simulink model "ACDCMG_sim8"  (R2022a)
settings: Solver=FixedStepAuto  StartTime=0.0  StopTime=0.5  FixedStep=Ts  MaxStep=1e-2  RelTol=1e-3
InitFcn:
  | Set_parameters_R2018
values from neighbouring files (symbols this model uses):
  D_invs = 0.05    [Set_parameters_R2018.m]
  dis11 = 3    [Set_parameters_R2018.m]
  dis12 = 3    [Set_parameters_R2018.m]
  dis2 = 0.2    [Set_parameters_R2018.m]
  dis3 = 0.15    [Set_parameters_R2018.m]
  dis4 = 0.2    [Set_parameters_R2018.m]
  dis5 = 0.25    [Set_parameters_R2018.m]
  dis6 = 0.1    [Set_parameters_R2018.m]
  Fnom = 60    [Set_parameters_R2018.m]
  H_invs = 6    [Set_parameters_R2018.m]
  max_min = 1    [Set_parameters_R2018.m]
  P_Load_3 = S_Load_3* PF_Load_3    (= 7650)    [Set_parameters_R2018.m]
  P_nom_inv = 3e3    (= 3000)    [Set_parameters_R2018.m]
  Pnom_T1 = 1.5e6    (= 1500000)    [Set_parameters_R2018.m]
  Pnom_T2 = 1.5e6    (= 1500000)    [Set_parameters_R2018.m]
  Pnom_T3 = 4e6    (= 4000000)    [Set_parameters_R2018.m]
  Ql_Load_3 = S_Load_3 * sin(acos(PF_Load_3))    [Set_parameters_R2018.m]
  R_Load_9 = (Vnom_prim * 1.35)^2 / P_Load_9    (= 1084.6153125)    [Set_parameters_R2018.m]
  R_Load_DC = Vnom_DC^2/ P_Load_DC    (= 45)    [Set_parameters_R2018.m]
  Rl = 0.17    [Set_parameters_R2018.m]
  Rls = 0.013    [Set_parameters_R2018.m]
  Ts = Ts_Power    (= 6.94444444444e-06)    [Set_parameters_R2018.m]
  Ts_Control = 6*Ts_Power    (= 4.16666666667e-05)    [Set_parameters_R2018.m]
  Ts_Inv = 0.07    [Set_parameters_R2018.m]
  Ts_Power = 1/(24*Fnom)/100    (= 6.94444444444e-06)    [Set_parameters_R2018.m]
  Ts_PV = 0.05    [Set_parameters_R2018.m]
  V1_LL_T3 = 69e3    (= 69000)    [Set_parameters_R2018.m]
  Vmin_mppt = 100    [Set_parameters_R2018.m]
  Vnom_DC = 300    [Set_parameters_R2018.m]
  Vnom_Diesel = 2.4e3    (= 2400)    [Set_parameters_R2018.m]
  Vnom_prim = 13.8e3    (= 13800)    [Set_parameters_R2018.m]
  Vnom_sec = 220    [Set_parameters_R2018.m]
  Vnom_ter_AC_DC = 150    [Set_parameters_R2018.m]
  Xl = 0.3    [Set_parameters_R2018.m]
  Xls = 0.93e-3    (= 0.00093)    [Set_parameters_R2018.m]
undefined symbols (not defined in the file or in its folder): D1, dEgdT, Delta, DiscIntNeverNeededParam, EgRef, fn, gcbh, Ion, k1, Lithium, Rsh_array5pc, sps_rtmsupport, Tref_K, VnInv, VT_ref
libraries: spsCurrentMeasurementLib x40, spsRMSLib x29, spsSeriesRLCBranchLib x23, spsVoltageMeasurementLib x21, spsMeanLib x14, spsThreePhaseVIMeasurementLib x14, powerlib_extras x13, spsThreePhaseSeriesRLCBranchLib x12, spsPower3phInstantaneousLib x10, spsBreakerLib x8, spsControlledVoltageSourceLib x8, spsPowerLib x8
(part 1 of 12)
settings Model: Creator=Leony  LastModifiedBy=dkh20
settings SolverCC: ZeroCrossAlgorithm=Adaptive  SolverResetMethod=Robust
settings DataIOCC: LimitDataPoints=on  SaveFormat=Array  ReturnWorkspaceOutputs=off
settings OptimizationCC: LifeSpan=inf
settings DebuggingCC: AlgebraicLoopMsg=none  UnderspecifiedInitializationDetection=Classic  MergeDetectMultiDrivingBlocksExec=none  IgnoredZcDiagnostic=none  SolverPrmCheckMsg=warning  UnconnectedInputMsg=warning  UnconnectedOutputMsg=warning  UnconnectedLineMsg=warning  AllowSymbolicDim=off  SFUnexpectedBacktrackingDiag=warning  SFNoUnconditionalDefaultTransitionDiag=warning  SFExecutionAtInitializationDiag=none  SFMachineParentedDataDiag=warning  ArithmeticOperatorsInVariantConditions=warning
settings HardwareCC: ProdBitPerPointer=32  ProdBitPerSizeT=32  ProdBitPerPtrDiffT=32  ProdLargestAtomicFloat=None  ProdIntDivRoundTo=Undefined  ProdEndianess=Unspecified  ProdWordSize=32  ProdHWDeviceType=32-bit Generic
settings ModelReferenceCC: PropagateSignalLabelsOutOfModel=off
settings SFSimCC: SimUseLocalCustomCode=off  CustomCodeUndefinedFunction=UseInterfaceOnly
settings RTWCC: RTWUseLocalCustomCode=off  DLArmComputeVersion=19.05
settings CodeAppCC: StateflowObjectComments=on
settings GRTTargetCC: TargetLangStandard=C89/C90 (ANSI)
settings ConfigComp: CovMetricSettings=dw  CovSaveCumulativeToWorkspaceVar=on  CovSaveSingleToWorkspaceVar=on  CovExternalEMLEnable=off
settings SimscapeCC: SimscapeNormalizeSystem=off

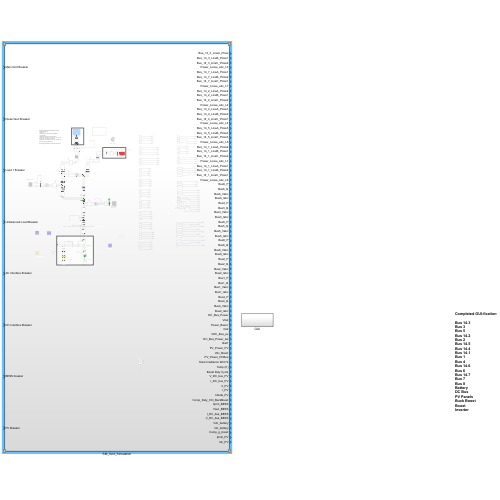
[thumbnail: Simulink's stored preview of the top-level diagram]
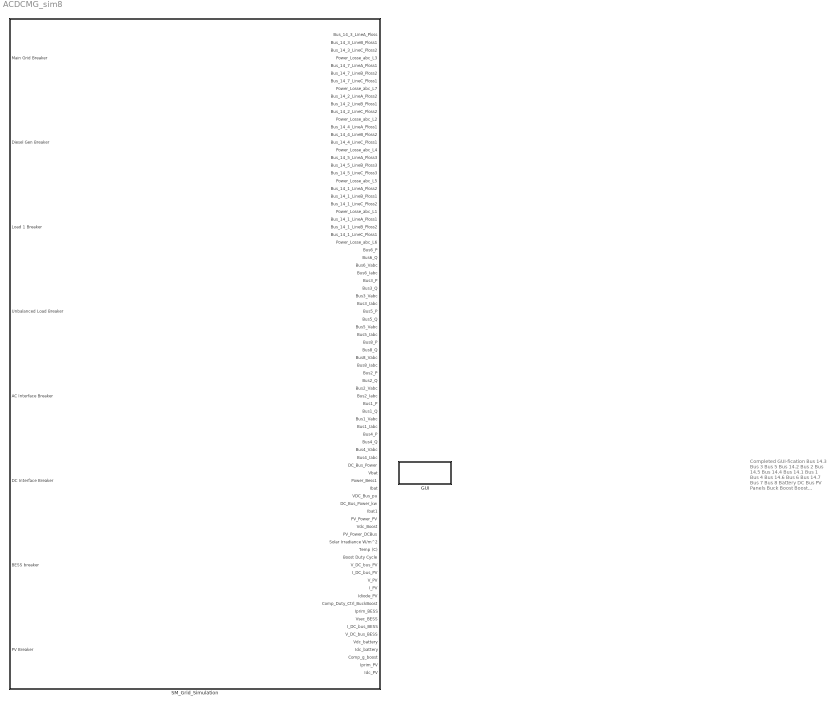
== system ACDCMG_sim8 ==
  note: Completed GUI-fication
      |
      | Bus 14.3
      | Bus 3
      | Bus 5
      | Bus 14.2
      | Bus 2
      | Bus 14.5
      | Bus 14.4
      | Bus 14.1
      | Bus 1
      | Bus 4
      | Bus 14.6
      | Bus 6
      | Bus 14.7
      | Bus 7
      | Bus 8
      | Battery
      | DC Bus
      | PV Panels
      | Buck Boost
      | Boost
      | Inverter
  GUI : Subsystem
  SM_Grid_Simulation : Subsystem

== system ACDCMG_sim8/GUI ==

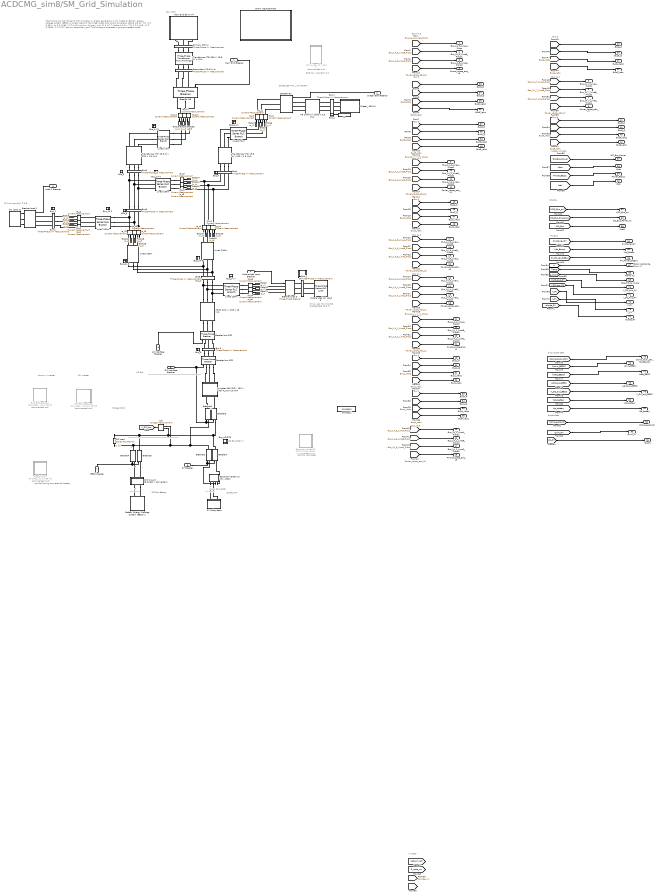
== system ACDCMG_sim8/SM_Grid_Simulation ==
  note: 9 kVA; cos (phi) = 0.85
      | Unbalanced 12.6 %
  note: +
  note: +
  note: Main Grid
  note: ---------------------------------------------------------------------------
  note: 2 kW
  note: +
  note: ---------------
  note: VF inverter
  note: DC Bus 300V V
  note: Microgrid DC
  note: Diesel_50 MVA _ Sim BusPV
  note: dump converter
  note: --------------------------------------------------------------------------------
  note: dummy converter
  note: dummy inverter
  note: ---------------
  note: -
  note: 12 kVA; cos (phi) = 0.6
  note: -
  note: DC Bus PV
  note: -
  note: DC Bus Battery
  note: The Hybrid AC /DC Microgrid (MG) includes:
      | 1- Diesel generators
      | 2- PV model
      | 3- Battery energy storage system (BESS)
      | 4- Linear loads
      | 5- Nonlinear loads such as arc furnace
      | 6- Cable 1/0 Cu, TW. R = 0.394 / XL = 0.1168 / Z = 0.411 per km. (Primary grid 13.8 kV)
      | 7- Cable 4/0 Cu , TW R = 0.198 / Xl = 0.1089 / Z = 0.227 per km (secondary grid)
      |
      | The microgrid operates in grid-connected mode.
  note: grid-following converter for battery
  note: +
  note: 320 kVA ; cos (phi) = 1
  note: AC Bus
  note: +
  note: -
  note: -
  note: inverter
  note: Bus 1
  note: Bus 14.4
  note: Bus 4
  note: Bus 5
  note: Bus 14.5
  note: Bus 14.6
  note: Bus 2
  note: Bus 3
  note: Bus 14.1
  note: Bus 14.2
  note: Bus 14.3
  note: Bus 8
  note: Bus 6
  note: DC_Bus
  note: PV_Bus
  note: buck boost data
  note: Bus 14.7
  note: battery_system
  note: boost data
  Main Grid Breaker : Inport
  Diesel Gen Breaker : Inport  Port=2
  Load 1 Breaker : Inport  Port=3
  Unbalanced Load Breaker : Inport  Port=4
  AC Interface Breaker : Inport  Port=5
  DC Interface Breaker : Inport  Port=6
  BESS breaker : Inport  Port=7
  PV Breaker : Inport  Port=8
    Ic_L{1,3..4,11} (4 alike) : spsCurrentMeasurementLib/Current Measurement  PhasorSimulation=off  OutputType=Complex  PSBequivalent=0
  AC  Load 11 : spsThreePhaseSeriesRLCLoadLib/Three-Phase Series RLC Load  LConnTagsString=A|B|C  Configuration=Y (grounded)  NominalVoltage=Vnom_sec  Vabc=[1e3 1e3 1e3]  Vabcp=[1e3 1e3 1e3]  NominalFrequency=Fnom  UnbalancedPower=off  ActivePower=P_Load_11  InductivePower=Ql_Load_11  CapacitivePower=0  Pabc=[10e3 9e3 11e3]  QLabc=[100 90 110]  QCabc=[100 90 110]  Pabcp=[10e3 9e3 11e3]  QLabcp=[100 90 110]  QCabcp=[100 90 110]  Measurements=None  LoadType=constant Z
  Battery Energy Storage System (BESS) 1 : Subsystem
      mask Display: image('Icons\Battery Energy Storage System (BESS).png');
  Boost -buck Bi-directional converter 1 : Subsystem
      mask Display: image(imread('Icons\DC_DC_Converter.jpg'));
  Boost -buck Bi-directional converter DC /CD 1 0.65 kW : Subsystem  Commented=on
      mask Display: image(imread('Icons\DC_DC_Converter.jpg'));
  "Boost converter 2 5 kHz - 300V " : Subsystem
      mask Display: image(imread('Icons\DC_DC_Converter.jpg'));
  "Boost converter DC /DC 2 5 kHz - 300V " : Subsystem  Commented=on
      mask Display: image(imread('Icons\DC_DC_Converter.jpg'));
  Breaker G1 : spsThreePhaseBreakerLib/Three-Phase Breaker  InitialState=closed  SwitchA=on  SwitchB=on  SwitchC=on  SwitchTimes="[4/60  10/60]"  External=on  BreakerResistance=0.001  SnubberResistance=1e6  SnubberCapacitance=inf  Measurements=None
  Breaker Load 1 : spsThreePhaseBreakerLib/Three-Phase Breaker  InitialState=closed  SwitchA=on  SwitchB=on  SwitchC=on  SwitchTimes="[4/60  10/60]"  External=on  BreakerResistance=0.001  SnubberResistance=1e6  SnubberCapacitance=inf  Measurements=None
  Breaker Load 3 : spsThreePhaseBreakerLib/Three-Phase Breaker  InitialState=closed  SwitchA=on  SwitchB=on  SwitchC=on  SwitchTimes="[4/60  10/60]"  External=on  BreakerResistance=0.001  SnubberResistance=1e6  SnubberCapacitance=inf  Measurements=None
  Breaker MG : spsThreePhaseBreakerLib/Three-Phase Breaker  InitialState=closed  SwitchA=on  SwitchB=on  SwitchC=on  SwitchTimes="[4/60  10/60]"  External=on  BreakerResistance=0.001  SnubberResistance=1e6  SnubberCapacitance=inf  Measurements=None
  Breaker bus DC1 : spsThreePhaseBreakerLib/Three-Phase Breaker  InitialState=closed  SwitchA=on  SwitchB=on  SwitchC=on  SwitchTimes="[4/60  10/60]"  External=on  BreakerResistance=0.001  SnubberResistance=1e6  SnubberCapacitance=inf  Measurements=None
  Breaker bus DC2 : spsThreePhaseBreakerLib/Three-Phase Breaker  InitialState=closed  SwitchA=on  SwitchB=on  SwitchC=on  SwitchTimes="[4/60  10/60]"  External=on  BreakerResistance=0.001  SnubberResistance=1e6  SnubberCapacitance=inf  Measurements=None
  Breaker{2..5} (4 alike) : spsBreakerLib/Breaker  InitialState=1  SwitchingTimes="[1/60  5/60]"  External=on  BreakerResistance=0.01  SnubberResistance=1e6  SnubberCapacitance=inf  Measurements=None  MoreParameters=on  NoBreakLoop=off
      settings: SourceProductBaseCode=PS
  Breaker6 : spsBreakerLib/Breaker  InitialState=0  SwitchingTimes="[1/60  5/60]"  External=on  BreakerResistance=0.01  SnubberResistance=1e6  SnubberCapacitance=inf  Measurements=None  MoreParameters=on  NoBreakLoop=off
      settings: SourceProductBaseCode=PS
  Breaker7 : spsBreakerLib/Breaker  InitialState=0  SwitchingTimes="[1/60  5/60]"  External=on  BreakerResistance=0.01  SnubberResistance=1e6  SnubberCapacitance=inf  Measurements=None  MoreParameters=on  NoBreakLoop=off
      settings: SourceProductBaseCode=PS
  Bus 1 : spsThreePhaseVIMeasurementLib/Three-Phase V-I Measurement  VoltageMeasurement=phase-to-phase  SetLabelV=on  LabelV=VabcLL_Bus_1  Vpu=off  VpuLL=off  CurrentMeasurement=yes  SetLabelI=on  LabelI=IabcLL_Bus_1  Ipu=off  Pbase=100e6  Vbase=25e3/sqrt(2)  OutputType=Complex  PhasorSimulation=off  PSBequivalent=0
  Bus 2 : spsThreePhaseVIMeasurementLib/Three-Phase V-I Measurement  VoltageMeasurement=phase-to-phase  SetLabelV=on  LabelV=VabcLL_Bus_2  Vpu=off  VpuLL=off  CurrentMeasurement=yes  SetLabelI=on  LabelI=IabcLL_Bus_2  Ipu=off  Pbase=100e6  Vbase=380/sqrt(2)  OutputType=Complex  PhasorSimulation=off  PSBequivalent=0
  Bus 7 : spsThreePhaseVIMeasurementLib/Three-Phase V-I Measurement  VoltageMeasurement=phase-to-phase  SetLabelV=on  LabelV=VabcLL_Bus_7  Vpu=off  VpuLL=off  CurrentMeasurement=yes  SetLabelI=on  LabelI=IabcLL_Bus_7  Ipu=off  Pbase=100e6  Vbase=380/sqrt(2)  OutputType=Complex  PhasorSimulation=off  PSBequivalent=0
  Bus 8 : spsThreePhaseVIMeasurementLib/Three-Phase V-I Measurement  VoltageMeasurement=phase-to-phase  SetLabelV=on  LabelV=VabcLL_Bus_8  Vpu=off  VpuLL=off  CurrentMeasurement=yes  SetLabelI=on  LabelI=IabcLL_Bus_8  Ipu=off  Pbase=100e6  Vbase=25e3  OutputType=Complex  PhasorSimulation=off  PSBequivalent=0
  Bus3 : spsThreePhaseVIMeasurementLib/Three-Phase V-I Measurement  VoltageMeasurement=phase-to-phase  SetLabelV=on  LabelV=VabcLL_Bus_3  Vpu=off  VpuLL=off  CurrentMeasurement=yes  SetLabelI=on  LabelI=IabcLL_Bus_3  Ipu=off  Pbase=100e6  Vbase=380/sqrt(2)  OutputType=Complex  PhasorSimulation=off  PSBequivalent=0
  Bus4 : spsThreePhaseVIMeasurementLib/Three-Phase V-I Measurement  VoltageMeasurement=phase-to-phase  SetLabelV=on  LabelV=VabcLL_Bus_4  Vpu=off  VpuLL=off  CurrentMeasurement=yes  SetLabelI=on  LabelI=IabcLL_Bus_4  Ipu=off  Pbase=100e6  Vbase=380/sqrt(2)  OutputType=Complex  PhasorSimulation=off  PSBequivalent=0
  Bus5 : spsThreePhaseVIMeasurementLib/Three-Phase V-I Measurement  VoltageMeasurement=phase-to-phase  SetLabelV=on  LabelV=VabcLL_Bus_5  Vpu=off  VpuLL=off  CurrentMeasurement=yes  SetLabelI=on  LabelI=IabcLL_Bus_5  Ipu=off  Pbase=100e6  Vbase=380/sqrt(2)  OutputType=Complex  PhasorSimulation=off  PSBequivalent=0
  Bus6 : spsThreePhaseVIMeasurementLib/Three-Phase V-I Measurement  VoltageMeasurement=phase-to-phase  SetLabelV=on  LabelV=VabcLL_Bus_6  Vpu=off  VpuLL=off  CurrentMeasurement=yes  SetLabelI=on  LabelI=IabcLL_Bus_6  Ipu=off  Pbase=100e6  Vbase=380/sqrt(2)  OutputType=Complex  PhasorSimulation=off  PSBequivalent=0
  Bus_1 : Subsystem
  Bus_14 1 : Subsystem
  Bus_14 2 : Subsystem
  Bus_14 3 : Subsystem
  Bus_14 4 : Subsystem
  Bus_14 5 : Subsystem
  Bus_14 6 : Subsystem
  Bus_14 7 : Subsystem
  Bus_2 : Subsystem
  Bus_3 : Subsystem
  Bus_4 : Subsystem
  Bus_5 : Subsystem
  Bus_6 : Subsystem
  Bus_7 : Subsystem
      mask Display: image('Icons\S_meeter.png');
  Bus_8 : Subsystem
  Bus_AC/DC3 : Subsystem
  DATA  ADQUISITION : Subsystem
      mask Display: image('Icons\SCADA.png');
  DC Load : spsSeriesRLCBranchLib/Series RLC Branch  LConnTagsString=__new0  RConnTagsString=__new0  BranchType=R  Resistance=R_Load_DC  Inductance=1e-3  SetiL0=off  InitialCurrent=0  Capacitance=1e-6  Setx0=off  InitialVoltage=0  Measurements=None
  Diesel_ 50MVA : Subsystem
      mask Display: image(imread('Icons\Diesel 50kW1.png'));
  Grid Bi-directional Converter 1.1 300 (DC) / 150 V (AC) P_nom 3kW2 : Subsystem  Commented=on
      mask Display: image(imread('Icons\Inverter.png'));
  Grid Bi-directional Converter 1.2 300 (DC) / 150 V (AC) P_nom 3kW3 : Subsystem  Commented=on
      mask Display: image(imread('Icons\Inverter.png'));
  Ia_L{1..6,11} (7 alike) : spsCurrentMeasurementLib/Current Measurement  PhasorSimulation=off  OutputType=Complex  PSBequivalent=0
  Ib_L{1..6,11} (7 alike) : spsCurrentMeasurementLib/Current Measurement  PhasorSimulation=off  OutputType=Complex  PSBequivalent=0
  Ic_L2 : spsCurrentMeasurementLib/Current Measurement  PhasorSimulation=off  OutputType=Complex  PSBequivalent=0
  Ic_L5 : spsCurrentMeasurementLib/Current Measurement  PhasorSimulation=off  OutputType=Complex  PSBequivalent=0
  Ic_L6 : spsCurrentMeasurementLib/Current Measurement  PhasorSimulation=off  OutputType=Complex  PSBequivalent=0
  Inverter 300 (DC) / 150 V (AC) P_nom 10 kW4 : Subsystem
      mask Display: image('Icons\Inverter.png'); % Use "Edit Image" on toolstrip to change.
  Line11 3km : spsThreePhaseSeriesRLCBranchLib/Three-Phase Series RLC Branch  LConnTagsString=A|B|C  RConnTagsString=A|B|C  BranchType=RL  Resistance=Rl* dis11  Inductance=Xl/377 * dis11  Capacitance=1e-6  Measurements=None
  Line12 3km : spsThreePhaseSeriesRLCBranchLib/Three-Phase Series RLC Branch  LConnTagsString=A|B|C  RConnTagsString=A|B|C  BranchType=RL  Resistance=Rl* dis12  Inductance=Xl/377 * dis12  Capacitance=1e-6  Measurements=None
  Line2 200m : spsThreePhaseSeriesRLCBranchLib/Three-Phase Series RLC Branch  LConnTagsString=A|B|C  RConnTagsString=A|B|C  BranchType=RL  Resistance=Rls * dis2  Inductance=Xls/377 * dis2  Capacitance=1e-6  Measurements=None
  Line3 150m : spsThreePhaseSeriesRLCBranchLib/Three-Phase Series RLC Branch  LConnTagsString=A|B|C  RConnTagsString=A|B|C  BranchType=RL  Resistance=Rls * dis3  Inductance=Xls/377 * dis3  Capacitance=1e-6  Measurements=None
  Line4 200m : spsThreePhaseSeriesRLCBranchLib/Three-Phase Series RLC Branch  LConnTagsString=A|B|C  RConnTagsString=A|B|C  BranchType=RL  Resistance=Rls * dis4  Inductance=Xls/377 * dis4  Capacitance=1e-6  Measurements=None
  Line5 250m : spsThreePhaseSeriesRLCBranchLib/Three-Phase Series RLC Branch  LConnTagsString=A|B|C  RConnTagsString=A|B|C  BranchType=RL  Resistance=Rls * dis5  Inductance=Xls/377 * dis5  Capacitance=1e-6  Measurements=None
  Line6 100m : spsThreePhaseSeriesRLCBranchLib/Three-Phase Series RLC Branch  LConnTagsString=A|B|C  RConnTagsString=A|B|C  BranchType=RL  Resistance=Rls * dis6  Inductance=Xls/377 * dis6  Capacitance=1e-6  Measurements=None
  Main Grid 69 kV Inf : Subsystem
      mask Display: image('Icons\Main-grid.png');
  Non Linear AC  Load 9 : Subsystem  Commented=on
  PV Subsystem : Subsystem
  Primary (69 kV) : spsThreePhaseVIMeasurementLib/Three-Phase V-I Measurement  VoltageMeasurement=phase-to-phase  SetLabelV=on  LabelV=Vabc_Prim_pu  Vpu=off  VpuLL=on  CurrentMeasurement=yes  SetLabelI=on  LabelI=Iabc_Prim_pu  Ipu=off  Pbase=10000e6  Vbase=69e3/sqrt(2)  OutputType=Magnitude  PhasorSimulation=off  PSBequivalent=0
  Secundario 13.8 kV LL : spsThreePhaseVIMeasurementLib/Three-Phase V-I Measurement  VoltageMeasurement=phase-to-phase  SetLabelV=on  LabelV=Vabc_Sec_pu  Vpu=off  VpuLL=on  CurrentMeasurement=yes  SetLabelI=on  LabelI=Iabc_Sec  Ipu=off  Pbase=250e6  Vbase=Vnom_prim/sqrt(2)  OutputType=Magnitude  PhasorSimulation=off  PSBequivalent=0
  TDC2 220 V / 150 V 15 kVA : spsThreePhaseTransformerTwoWindingsLib/Three-Phase Transformer (Two Windings)  Winding1Connection=Y  Winding2Connection=Y  CoreType=Three single-phase transformers  SetSaturation=off  Hysteresis=off  DataFile='hysteresis'  SetInitialFlux=off  Measurements=None  UNITS=pu  NominalPower=[15e3 , Fnom ]  Winding1=[Vnom_sec , 0.03/2 , 0.03/377 ]  Winding2=[Vnom_ter_AC_DC , 0.03/2 , 0.03/377 ]  Rm=500  Lm=500  L0=0.5  Saturation=[ 0,0 ; 0.0024,1.2 ; 1.0,1.52 ]  InitialFluxes=[ 0.8 , -0.8 , 0.7 ]  BreakLoop=off  DiscreteSolver=Trapezoidal iterative  DataType=off  TransfoNumber=1
  TG 13.8 kV / 2400 V 3.5 MVA : spsThreePhaseTransformerTwoWindingsLib/Three-Phase Transformer (Two Windings)  Winding1Connection=Yg  Winding2Connection=Delta (D1)  CoreType=Three single-phase transformers  SetSaturation=off  Hysteresis=off  DataFile='hysteresis'  SetInitialFlux=off  Measurements=None  UNITS=pu  NominalPower=[3.5e6 , Fnom ]  Winding1=[ Vnom_prim , 0.015/2 , 0.015/2/377]  Winding2=[ Vnom_Diesel , 0.015/2 , 0.015/2/377]  Rm=500  Lm=500  L0=0.5  Saturation="[ 0,0  ;  0.005,1.2  ;  1.0,1.4 ]"  InitialFluxes=[ 0.8 , -0.8 , 0.7 ]  BreakLoop=off  DiscreteSolver=Trapezoidal iterative  DataType=off  TransfoNumber=0
  Transformer (T1) 13.8 kV / 220 V 1.5 MVA : spsThreePhaseTransformerTwoWindingsLib/Three-Phase Transformer (Two Windings)  Winding1Connection=Y  Winding2Connection=Y  CoreType=Three single-phase transformers  SetSaturation=off  Hysteresis=off  DataFile='hysteresis'  SetInitialFlux=off  Measurements=None  UNITS=pu  NominalPower=[ Pnom_T1, Fnom ]  Winding1=[Vnom_prim , 0.03/2 , 0.03/(2*377) ]  Winding2=[Vnom_sec , 0.03/2 , 0.03/(2*377) ]  Rm=500  Lm=500  L0=0.5  Saturation=[ 0,0 ; 0.0024,1.2 ; 1.0,1.52 ]  InitialFluxes=[ 0.8 , -0.8 , 0.7 ]  BreakLoop=off  DiscreteSolver=Trapezoidal iterative  DataType=off  TransfoNumber=1
  Transformer (T2) 13.8 kV / 220 V 1.5 MVA : spsThreePhaseTransformerTwoWindingsLib/Three-Phase Transformer (Two Windings)  Winding1Connection=Y  Winding2Connection=Y  CoreType=Three single-phase transformers  SetSaturation=off  Hysteresis=off  DataFile='hysteresis'  SetInitialFlux=off  Measurements=None  UNITS=pu  NominalPower=[Pnom_T2 , Fnom]  Winding1=[ Vnom_prim, 0.03/2 , 0.03/(2*377) ]  Winding2=[Vnom_sec , 0.03/2 , 0.03/(2*377) ]  Rm=500  Lm=500  L0=0.5  Saturation=[ 0,0 ; 0.0024,1.2 ; 1.0,1.52 ]  InitialFluxes=[ 0.8 , -0.8 , 0.7 ]  BreakLoop=off  DiscreteSolver=Trapezoidal iterative  DataType=off  TransfoNumber=1
  Transformer (T3) 69kV / 13.8 kV 4 MVA : spsThreePhaseTransformerTwoWindingsLib/Three-Phase Transformer (Two Windings)  Winding1Connection=Yg  Winding2Connection=Delta (D1)  CoreType=Three single-phase transformers  SetSaturation=off  Hysteresis=off  DataFile='hysteresis'  SetInitialFlux=off  Measurements=None  UNITS=pu  NominalPower=[Pnom_T3 , Fnom ]  Winding1=[V1_LL_T3 , 0.015/2 , 0.015/(2*377)]  Winding2=[ Vnom_prim, 0.015/2 , 0.015/(2*377)]  Rm=500  Lm=500  L0=0.5  Saturation="[ 0,0  ;  0.005,1.2  ;  1.0,1.4 ]"  InitialFluxes=[ 0.8 , -0.8 , 0.7 ]  BreakLoop=off  DiscreteSolver=Trapezoidal iterative  DataType=off  TransfoNumber=0
  Unbalanced AC  Load 3 : spsThreePhaseSeriesRLCLoadLib/Three-Phase Series RLC Load  LConnTagsString=A|B|C  Configuration=Y (grounded)  NominalVoltage=Vnom_sec  Vabc=[Vnom_sec/sqrt(3), Vnom_sec/sqrt(3), Vnom_sec/sqrt(3)]  Vabcp=[1e3 1e3 1e3]  NominalFrequency=Fnom  UnbalancedPower=on  ActivePower=P_Load_3  InductivePower=Ql_Load_3  CapacitivePower=0  Pabc=[P_Load_3*1.04, P_Load_3, P_Load_3*0.9]  QLabc=[Ql_Load_3*1.04, Ql_Load_3, Ql_Load_3*0.9]  QCabc=[0 0 0]  Pabcp=[10e3 9e3 11e3]  QLabcp=[100 90 110]  QCabcp=[100 90 110]  Measurements=None  LoadType=constant Z
  "Vdc " : spsVoltageMeasurementLib/Voltage Measurement  Tag=PoWeRsYsTeMmEaSuReMeNt  PhasorSimulation=off  OutputType=Magnitude  PSBequivalent=0
  f1 : ToWorkspace  VariableName=Means_Bus1  SaveFormat=Timeseries  SampleTime=-1
  powergui : spspowerguiLib/powergui  Priority=1  SimulationMode=Discrete  SampleTime=Ts_Power  frequency=60  Iterations=50  frequencyindice=0  Pbase=100e6  ErrMax=1e-4  UnitsV=kV  UnitsW=MW  buscounter=0  FunctionMessages=off  echomessages=off  EnableUseOfTLC=off  CurrentSourceSwitches=off  DisableSnubberDevices=off  DisableRonSwitches=off  DisableVfSwitches=off  DisplayEquations=off  AutomaticDiscreteSolvers=off  SolverType=Tustin  Interpol=off  ExternalGateDelay=off  methode=off  Ts=0  x0status=blocks  SPID=off  SwTol=0  HookPort=off  NonlinearTolerance=1e-4  nMaxIteration=100  ContinueOnMaxIteration=off  RestoreLinks=warning  ResistiveCurrentMeasurement=off  Frange=[0:2:500]  Ylog=off  Xlog=on  ShowGrid=off  save=off  variable=ZData  structure=0  ZoomFFT=off  StartTime=0.0  cycles=1  DisplayStyle=1  fundamental=60  FreqAxis=off  MaxFrequency=1000  frequencyindicesteady=1  RmsSteady=1  display=off
  Bus_14_3_LineA_Ploss : Outport
  Bus_14_3_LineB_Ploss1 : Outport  Port=2
  Bus_14_3_LineC_Ploss2 : Outport  Port=3
  Power_Losse_abc_L3 : Outport  Port=4
  Bus_14_7_LineA_Ploss1 : Outport  Port=5
  Bus_14_7_LineB_Ploss2 : Outport  Port=6
  Bus_14_7_LineC_Ploss1 : Outport  Port=7
  Power_Losse_abc_L7 : Outport  Port=8
  Bus_14_2_LineA_Ploss2 : Outport  Port=9
  Bus_14_2_LineB_Ploss1 : Outport  Port=10
  Bus_14_2_LineC_Ploss2 : Outport  Port=11
  Power_Losse_abc_L2 : Outport  Port=12
  Bus_14_4_LineA_Ploss1 : Outport  Port=13
  Bus_14_4_LineB_Ploss2 : Outport  Port=14
  Bus_14_4_LineC_Ploss1 : Outport  Port=15
  Power_Losse_abc_L4 : Outport  Port=16
  Bus_14_5_LineA_Ploss3 : Outport  Port=17
  Bus_14_5_LineB_Ploss3 : Outport  Port=18
  Bus_14_5_LineC_Ploss3 : Outport  Port=19
  Power_Losse_abc_L5 : Outport  Port=20
  Bus_14_1_LineA_Ploss2 : Outport  Port=21
  Bus_14_1_LineB_Ploss1 : Outport  Port=22
  Bus_14_1_LineC_Ploss2 : Outport  Port=23
  Power_Losse_abc_L1 : Outport  Port=24
  Bus_14_1_LineA_Ploss1 : Outport  Port=25
  Bus_14_1_LineB_Ploss2 : Outport  Port=26
  Bus_14_1_LineC_Ploss1 : Outport  Port=27
  Power_Losse_abc_L6 : Outport  Port=28
  Bus6_P : Outport  Port=29
  Bus6_Q : Outport  Port=30
  Bus6_Vabc : Outport  Port=31
  Bus6_Iabc : Outport  Port=32
  Bus3_P : Outport  Port=33
  Bus3_Q : Outport  Port=34
  Bus3_Vabc : Outport  Port=35
  Bus3_Iabc : Outport  Port=36
  Bus5_P : Outport  Port=37
  Bus5_Q : Outport  Port=38
  Bus5_Vabc : Outport  Port=39
  Bus5_Iabc : Outport  Port=40
  Bus8_P : Outport  Port=41
  Bus8_Q : Outport  Port=42
  Bus8_Vabc : Outport  Port=43
  Bus8_Iabc : Outport  Port=44
  Bus2_P : Outport  Port=45
  Bus2_Q : Outport  Port=46
  Bus2_Vabc : Outport  Port=47
  Bus2_Iabc : Outport  Port=48
  Bus1_P : Outport  Port=49
  Bus1_Q : Outport  Port=50
  Bus1_Vabc : Outport  Port=51
  Bus1_Iabc : Outport  Port=52
  Bus4_P : Outport  Port=53
  Bus4_Q : Outport  Port=54
  Bus4_Vabc : Outport  Port=55
  Bus4_Iabc : Outport  Port=56
  DC_Bus_Power : Outport  Port=57
  Vbat : Outport  Port=58
  Power_Bess1 : Outport  Port=59
  Ibat : Outport  Port=60
  VDC_Bus_pu : Outport  Port=61
  DC_Bus_Power_kw : Outport  Port=62
  Ibat1 : Outport  Port=63
  PV_Power_PV : Outport  Port=64
  Vdc_Boost : Outport  Port=65
  PV_Power_DCBus : Outport  Port=66
  Solar Irradiance W/m^2 : Outport  Port=67
  Temp (C) : Outport  Port=68
  Boost Duty Cycle : Outport  Port=69
  V_DC_bus_PV : Outport  Port=70
  I_DC_bus_PV : Outport  Port=71
  V_PV : Outport  Port=72
  I_PV : Outport  Port=73
  Idiode_PV : Outport  Port=74
  Comp_Duty_Ctrl_BuckBoost : Outport  Port=75
  Iprim_BESS : Outport  Port=76
  Vsec_BESS : Outport  Port=77
  I_DC_bus_BESS : Outport  Port=78
  V_DC_bus_BESS : Outport  Port=79
  Vdc_battery : Outport  Port=80
  Idc_battery : Outport  Port=81
  Comp_g_boost : Outport  Port=82
  Iprim_PV : Outport  Port=83
  Idc_PV : Outport  Port=84
  tag scope: Ia_L1=global, Ia_L2=global, Ia_L3=global, Ia_L4=global, Ia_L5=global, Ia_L6=global, Ia_L7=global, Ib_L1=global, Ib_L2=global, Ib_L3=global, Ib_L4=global, Ib_L5=global, Ib_L6=global, Ib_L7=global, Ic_L1=global, Ic_L2=global, Ic_L3=global, Ic_L4=global, Ic_L5=global, Ic_L6=global, Ic_L7=global, V_DC_bus=global
  wires:
  Unbalanced Load Breaker/1 -> Breaker Load 3/1
  Load 1 Breaker/1 -> Breaker Load 1/1
  BESS breaker/1 -> Breaker5/1, Breaker4/1
  Ib_L4/1 -> [Ib_L6]
  Ia_L6/1 -> [Ia_L7]
  "  Ic_L4"/1 -> [Ic_L6]
  Ia_L4/1 -> [Ia_L6]
  Ia_L11/1 -> [Ia_L3]
  Ia_L3/1 -> [Ia_L5]
  Ib_L11/1 -> [Ib_L3]
  Ib_L3/1 -> [Ib_L5]
  Ib_L6/1 -> [Ib_L7]
  Ic_L6/1 -> [Ic_L7]
  "  Ic_L3"/1 -> [Ic_L5]
  "Vdc "/1 -> [V_DC_bus]
  Bus_1/1("Means_Bus1      ") -> f1/1
  Ic_L2/1 -> [Ic_L2]
  AC Interface Breaker/1 -> Breaker bus DC2/1
  DC Interface Breaker/1 -> Breaker3/1, Breaker2/1, Breaker bus DC1/1
  Ic_L5/1 -> [Ic_L4]
  Main Grid Breaker/1 -> Breaker MG/1
  "  Ic_L1"/1 -> [Ia_L1]
  "  Ic_L11"/1 -> [Ic_L3]
  Ib_L1/1 -> [Ib_L1]
  Ib_L2/1 -> [Ib_L2]
  Ia_L1/1 -> [Ic_L1]
  PV Breaker/1 -> Breaker7/1, Breaker6/1
  Ib_L5/1 -> [Ib_L4]
  Ia_L5/1 -> [Ia_L4]
  Ia_L2/1 -> [Ia_L2]
  Diesel Gen Breaker/1 -> Breaker G1/1
  [Bus_14_3_LineA_Ploss] -> Bus_14_3_LineA_Ploss/1
  [Bus_14_3_LineB_Ploss] -> Bus_14_3_LineB_Ploss1/1
  [Bus_14_3_LineC_Ploss] -> Bus_14_3_LineC_Ploss2/1
  [Power_Losse_abc_L3] -> Power_Losse_abc_L3/1
  [Bus_14_7_LineB_Ploss] -> Bus_14_7_LineB_Ploss2/1
  [Bus_14_7_LineA_Ploss] -> Bus_14_7_LineA_Ploss1/1
  [Bus_14_7_LineC_Ploss] -> Bus_14_7_LineC_Ploss1/1
  [Power_Losse_abc_L7] -> Power_Losse_abc_L7/1
  [Power_Losse_abc_L2] -> Power_Losse_abc_L2/1
  [Bus_14_2_LineC_Ploss] -> Bus_14_2_LineC_Ploss2/1
  [Bus_14_2_LineA_Ploss] -> Bus_14_2_LineA_Ploss2/1
  [Bus_14_2_LineB_Ploss] -> Bus_14_2_LineB_Ploss1/1
  [Bus_14_4_LineB_Ploss] -> Bus_14_4_LineB_Ploss2/1
  [Bus_14_4_LineA_Ploss] -> Bus_14_4_LineA_Ploss1/1
  [Bus_14_4_LineC_Ploss] -> Bus_14_4_LineC_Ploss1/1
  [Power_Losse_abc_L4] -> Power_Losse_abc_L4/1
  [Power_Losse_abc_L5] -> Power_Losse_abc_L5/1
  [Bus_14_5_LineC_Ploss] -> Bus_14_5_LineC_Ploss3/1
  [Bus_14_5_LineA_Ploss] -> Bus_14_5_LineA_Ploss3/1
  [Bus_14_5_LineB_Ploss] -> Bus_14_5_LineB_Ploss3/1
  [Power_Losse_abc_L1] -> Power_Losse_abc_L1/1
  [Bus_14_1_LineC_Ploss] -> Bus_14_1_LineC_Ploss2/1
  [Bus_14_1_LineA_Ploss] -> Bus_14_1_LineA_Ploss2/1
  [Bus_14_1_LineB_Ploss] -> Bus_14_1_LineB_Ploss1/1
  [Bus_14_6_LineB_Ploss] -> Bus_14_1_LineB_Ploss2/1
  [Bus_14_6_LineA_Ploss] -> Bus_14_1_LineA_Ploss1/1
  [Bus_14_6_LineC_Ploss] -> Bus_14_1_LineC_Ploss1/1
  [Power_Losse_abc_L6] -> Power_Losse_abc_L6/1
  [Bus6_Iabc] -> Bus6_Iabc/1
  [Bus6_Vabc] -> Bus6_Vabc/1
  [Bus6_Q] -> Bus6_Q/1
  [Bus6_P] -> Bus6_P/1
  [Bus3_P] -> Bus3_P/1
  [Bus3_Q] -> Bus3_Q/1
  [Bus3_Iabc] -> Bus3_Vabc/1
  [Bus3_Vabc] -> Bus3_Iabc/1
  [Bus5_Vabc] -> Bus5_Vabc/1
  [Bus5_Q] -> Bus5_Q/1
  [Bus5_P] -> Bus5_P/1
  [Bus5_Iabc] -> Bus5_Iabc/1
  [Bus8_Iabc] -> Bus8_Iabc/1
  [Bus8_P] -> Bus8_P/1
  [Bus8_Q] -> Bus8_Q/1
  [Bus8_Vabc] -> Bus8_Vabc/1
  [Bus2_Iabc] -> Bus2_Iabc/1
  [Bus2_P] -> Bus2_P/1
  [Bus2_Q] -> Bus2_Q/1
  [Bus2_Vabc] -> Bus2_Vabc/1
  [Bus1_Vabc] -> Bus1_Vabc/1
  [Bus1_Q] -> Bus1_Q/1
  [Bus1_P] -> Bus1_P/1
  [Bus1_Iabc] -> Bus1_Iabc/1
  [Bus4_Iabc] -> Bus4_Iabc/1
  [Bus4_P] -> Bus4_P/1
  [Bus4_Q] -> Bus4_Q/1
  [Bus4_Vabc] -> Bus4_Vabc/1
  [Ibat] -> Ibat/1
  [DC_Bus_Power] -> DC_Bus_Power/1
  [Vbat] -> Vbat/1
  [Power_Bess1] -> Power_Bess1/1
  [DC_Bus_Power_kw] -> DC_Bus_Power_kw/1
  [VDC_Bus_pu] -> VDC_Bus_pu/1
  [IDC_Bus] -> Ibat1/1
  [PV_Power_DCBus] -> PV_Power_DCBus/1
  [PV_Power_PV] -> PV_Power_PV/1
  [Vdc_Boost] -> Vdc_Boost/1
  [Temp] -> Temp (C)/1
  [Ir] -> Solar Irradiance W/m^2/1
  [g_boost] -> Boost Duty Cycle/1  "Duty Cycle"
  [Idiode_PV] -> Idiode_PV/1
  [V_PV] -> V_PV/1
  [V_DC_bus_PV] -> V_DC_bus_PV/1
  [I_DC_bus_PV] -> I_DC_bus_PV/1
  [I_PV] -> I_PV/1
  [Comp_Duty_Ctrl] -> Comp_Duty_Ctrl_BuckBoost/1
  [Iprim_BESS] -> Iprim_BESS/1
  [Vsec_BESS] -> Vsec_BESS/1
  [I_DC_bus_BESS] -> I_DC_bus_BESS/1
  [V_DC_bus_BESS] -> V_DC_bus_BESS/1
  [Vdc_battery] -> Vdc_battery/1
  [Idc_battery] -> Idc_battery/1
  [Comp_g_boost] -> Comp_g_boost/1
  [Iprim_PV] -> Iprim_PV/1
  [Idc_PV] -> Idc_PV/1
  connections:
  DC Load/LConn1 -- Breaker4/RConn1 -- "Vdc "/LConn1 -- Breaker2/LConn1 -- Breaker6/RConn1
  Bus5/LConn2 -- Line5 250m/LConn2 -- Bus3/RConn2
  Line4 200m/LConn1 -- Line3 150m/LConn1 -- Bus6/RConn1
  Line4 200m/LConn2 -- Line3 150m/LConn2 -- Bus6/RConn2
  Bus5/LConn3 -- Line5 250m/LConn3 -- Bus3/RConn3
  Breaker7/RConn1 -- Breaker3/LConn1 -- "Vdc "/LConn2 -- DC Load/RConn1 -- Breaker5/RConn1
  TDC2 220 V / 150 V 15 kVA/LConn3 -- Line6 100m/LConn3 -- Bus6/LConn3
  Bus4/RConn2 -- Ib_L4/LConn1 -- Ib_L5/RConn1
  Line4 200m/LConn3 -- Line3 150m/LConn3 -- Bus6/RConn3
  Bus5/LConn1 -- Line5 250m/LConn1 -- Bus3/RConn1
  Bus4/RConn3 -- "  Ic_L4"/LConn1 -- Ic_L5/RConn1
  Bus4/RConn1 -- Ia_L4/LConn1 -- Ia_L5/RConn1
  Bus5/RConn3 -- "  Ic_L3"/LConn1 -- Line2 200m/RConn3
  Bus5/RConn1 -- Ia_L3/LConn1 -- Line2 200m/RConn1
  TDC2 220 V / 150 V 15 kVA/LConn2 -- Line6 100m/LConn2 -- Bus6/LConn2
  Bus5/RConn2 -- Ib_L3/LConn1 -- Line2 200m/RConn2
  TDC2 220 V / 150 V 15 kVA/LConn1 -- Line6 100m/LConn1 -- Bus6/LConn1
  Ia_L1/RConn1 -- Line12 3km/RConn3
  Bus 2/LConn2 -- Breaker Load 1/LConn2
  AC  Load 11/LConn3 -- Breaker Load 1/RConn3
  Line11 3km/LConn3 -- Transformer (T1) 13.8 kV / 220 V 1.5 MVA/LConn3
  Bus 8/RConn3 -- Breaker bus DC2/LConn3
  Boost -buck Bi-directional converter 1/RConn1 -- Breaker4/LConn1
  Unbalanced AC  Load 3/LConn3 -- Bus 7/RConn3
  Line12 3km/LConn2 -- Transformer (T2) 13.8 kV / 220 V 1.5 MVA/LConn2
  AC  Load 11/LConn2 -- Breaker Load 1/RConn2
  Breaker MG/LConn3 -- Secundario 13.8 kV LL/RConn3
  Breaker bus DC1/LConn2 -- Inverter 300 (DC) / 150 V (AC) P_nom 10 kW4/LConn2
  Breaker G1/RConn1 -- "  Ic_L1"/LConn1
  Diesel_ 50MVA/LConn2 -- Bus 1/LConn2
  TG 13.8 kV / 2400 V 3.5 MVA/LConn3 -- Breaker G1/LConn3
  Breaker Load 3/LConn3 -- Ic_L6/RConn1
  Bus 1/RConn2 -- TG 13.8 kV / 2400 V 3.5 MVA/RConn2
  TDC2 220 V / 150 V 15 kVA/RConn2 -- Breaker bus DC2/RConn2
  Transformer (T2) 13.8 kV / 220 V 1.5 MVA/RConn1 -- Bus4/LConn1
  Bus 7/LConn2 -- Breaker Load 3/RConn2
  Diesel_ 50MVA/LConn1 -- Bus 1/LConn1
  Diesel_ 50MVA/LConn3 -- Bus 1/LConn3
  Bus 1/RConn1 -- TG 13.8 kV / 2400 V 3.5 MVA/RConn1
  Line5 250m/RConn1 -- Ia_L5/LConn1
  Bus 1/RConn3 -- TG 13.8 kV / 2400 V 3.5 MVA/RConn3
  "Boost converter 2 5 kHz - 300V "/RConn4 -- Breaker7/LConn1
  TG 13.8 kV / 2400 V 3.5 MVA/LConn1 -- Breaker G1/LConn1
  Line3 150m/RConn3 -- "  Ic_L3"/RConn1
  Bus 7/LConn1 -- Breaker Load 3/RConn1
  Line5 250m/RConn3 -- Ic_L5/LConn1
  Primary (69 kV)/RConn2 -- Transformer (T3) 69kV / 13.8 kV 4 MVA/LConn2
  Line4 200m/RConn2 -- Ib_L4/RConn1
  Bus 2/RConn2 -- Ib_L2/RConn1
  Line11 3km/RConn3 -- "  Ic_L11"/RConn1
  Breaker Load 3/LConn2 -- Ib_L6/RConn1
  Line3 150m/RConn2 -- Ib_L3/RConn1
  Line4 200m/RConn1 -- Ia_L4/RConn1
  Line5 250m/RConn2 -- Ib_L5/LConn1
  Line2 200m/LConn3 -- Ic_L2/LConn1
  Bus 8/LConn1 -- Breaker bus DC1/RConn1
  Line6 100m/RConn3 -- Ic_L6/LConn1
  Bus 8/LConn2 -- Breaker bus DC1/RConn2
  Breaker Load 3/LConn1 -- Ia_L6/RConn1
  Primary (69 kV)/LConn3 -- Main Grid 69 kV Inf/RConn1
  Bus 2/RConn1 -- Ia_L2/RConn1
  Primary (69 kV)/LConn1 -- Main Grid 69 kV Inf/RConn3
  TDC2 220 V / 150 V 15 kVA/RConn3 -- Breaker bus DC2/RConn3
  Bus 8/RConn2 -- Breaker bus DC2/LConn2
  Bus 8/LConn3 -- Breaker bus DC1/RConn3
  Breaker G1/RConn2 -- Ib_L1/LConn1
  AC  Load 11/LConn1 -- Breaker Load 1/RConn1
  Boost -buck Bi-directional converter 1/RConn2 -- Breaker5/LConn1
  Transformer (T1) 13.8 kV / 220 V 1.5 MVA/RConn1 -- Bus3/LConn1
  Breaker bus DC1/LConn1 -- Inverter 300 (DC) / 150 V (AC) P_nom 10 kW4/LConn1
  Breaker MG/LConn1 -- Secundario 13.8 kV LL/RConn1
  Line11 3km/RConn1 -- Ia_L11/RConn1
  Unbalanced AC  Load 3/LConn1 -- Bus 7/RConn1
  Line3 150m/RConn1 -- Ia_L3/RConn1
  Line2 200m/LConn2 -- Ib_L2/LConn1
  Bus 2/RConn3 -- Ic_L2/RConn1
  Boost -buck Bi-directional converter 1/LConn2 -- Battery Energy Storage System (BESS) 1/LConn2
  Ib_L1/RConn1 -- Line12 3km/RConn2
  TG 13.8 kV / 2400 V 3.5 MVA/LConn2 -- Breaker G1/LConn2
  Transformer (T3) 69kV / 13.8 kV 4 MVA/RConn3 -- Secundario 13.8 kV LL/LConn3
  Transformer (T1) 13.8 kV / 220 V 1.5 MVA/RConn3 -- Bus3/LConn3
  Line11 3km/LConn1 -- Transformer (T1) 13.8 kV / 220 V 1.5 MVA/LConn1
  Line4 200m/RConn3 -- "  Ic_L4"/RConn1
  Breaker MG/RConn2 -- Ib_L11/LConn1
  "  Ic_L1"/RConn1 -- Line12 3km/RConn1
  Primary (69 kV)/RConn1 -- Transformer (T3) 69kV / 13.8 kV 4 MVA/LConn1
  Transformer (T3) 69kV / 13.8 kV 4 MVA/RConn2 -- Secundario 13.8 kV LL/LConn2
  Boost -buck Bi-directional converter 1/LConn1 -- Battery Energy Storage System (BESS) 1/LConn1
  Bus 2/LConn1 -- Breaker Load 1/LConn1
  Primary (69 kV)/LConn2 -- Main Grid 69 kV Inf/RConn2
  "Boost converter 2 5 kHz - 300V "/RConn3 -- Breaker6/LConn1
  Bus 8/RConn1 -- Breaker bus DC2/LConn1
  Breaker MG/RConn3 -- "  Ic_L11"/LConn1
  Bus 7/LConn3 -- Breaker Load 3/RConn3
  "Boost converter 2 5 kHz - 300V "/RConn2 -- PV Subsystem/RConn2
  Breaker3/RConn1 -- Inverter 300 (DC) / 150 V (AC) P_nom 10 kW4/RConn2
  Line6 100m/RConn1 -- Ia_L6/LConn1
  Transformer (T2) 13.8 kV / 220 V 1.5 MVA/RConn2 -- Bus4/LConn2
  Unbalanced AC  Load 3/LConn2 -- Bus 7/RConn2
  "Boost converter 2 5 kHz - 300V "/RConn1 -- PV Subsystem/RConn1
  Transformer (T2) 13.8 kV / 220 V 1.5 MVA/RConn3 -- Bus4/LConn3
  Line12 3km/LConn1 -- Transformer (T2) 13.8 kV / 220 V 1.5 MVA/LConn1
  Bus 2/LConn3 -- Breaker Load 1/LConn3
  Line11 3km/RConn2 -- Ib_L11/RConn1
  Line6 100m/RConn2 -- Ib_L6/LConn1
  Primary (69 kV)/RConn3 -- Transformer (T3) 69kV / 13.8 kV 4 MVA/LConn3
  Breaker bus DC1/LConn3 -- Inverter 300 (DC) / 150 V (AC) P_nom 10 kW4/LConn3
  Breaker2/RConn1 -- Inverter 300 (DC) / 150 V (AC) P_nom 10 kW4/RConn1
  Breaker MG/LConn2 -- Secundario 13.8 kV LL/RConn2
  Line11 3km/LConn2 -- Transformer (T1) 13.8 kV / 220 V 1.5 MVA/LConn2
  Line12 3km/LConn3 -- Transformer (T2) 13.8 kV / 220 V 1.5 MVA/LConn3
  TDC2 220 V / 150 V 15 kVA/RConn1 -- Breaker bus DC2/RConn1
  Transformer (T1) 13.8 kV / 220 V 1.5 MVA/RConn2 -- Bus3/LConn2
  Breaker G1/RConn3 -- Ia_L1/LConn1
  Breaker MG/RConn1 -- Ia_L11/LConn1
  Line2 200m/LConn1 -- Ia_L2/LConn1
  Transformer (T3) 69kV / 13.8 kV 4 MVA/RConn1 -- Secundario 13.8 kV LL/LConn1

== system ACDCMG_sim8/SM_Grid_Simulation/Battery Energy Storage System (BESS) 1 ==
  Battery1 : spsBatteryLib/Battery  BatType=Lithium-Ion  ShowTempParam=off  ThermalPreset=no  ShowAgeParam=off  NomV=120  NomQ=800  SOC=80  Batt_Tr=3  PresetModel=on  MaxQ=800  MinV=90  FullV=139.6785  Dis_rate=347.8261  R=0.0015  Normal_OP=723.4783  expZone="[129.6463      39.30435]"  current=[30 35 40 46]  Units=Time  Tci=20  NomT=25  T2=0  MaxQ2=2.208  FullV2=3.45  Normal_OP2=2.8  expZone2="[3.22        0.23]"  Rca=0.6  ti=1000  Dp=0  Neq0=0  Tsim=1e6  Ta1=25  Qeol=5.4*0.9  Reol=0.013333*1.2  Char_age=[2.3478, 3]  Dis_age=[2.3478, 10]  N1=1500  N2=10500  N3=1000  N4=1400  Ta2=45  N5=950
  + B1 : PMIOPort  Side=Left
  - B1 : PMIOPort  Port=2  Side=Left
  connections:
  Battery1/LConn2 -- - B1/RConn1
  Battery1/LConn1 -- + B1/RConn1

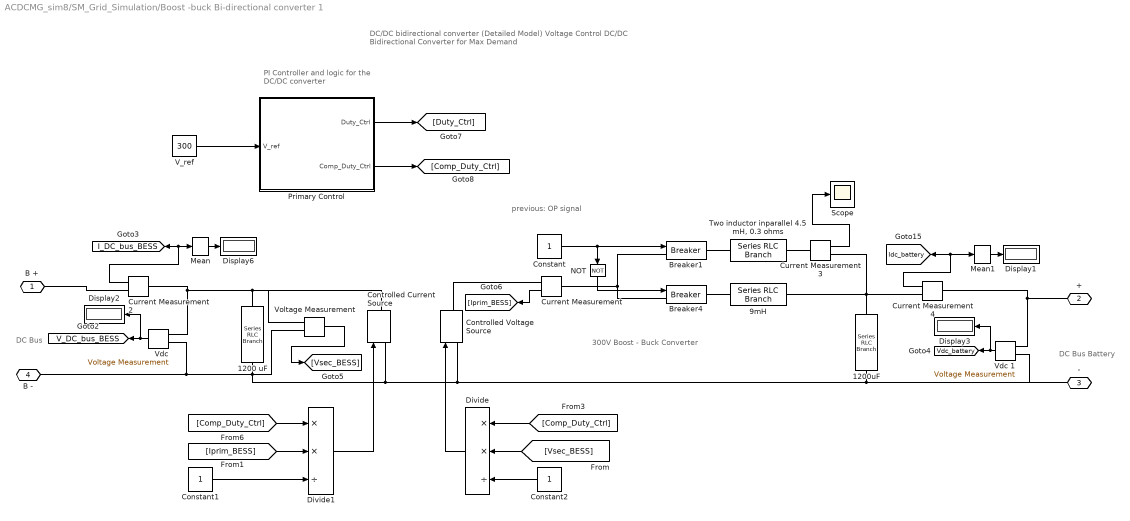
== system ACDCMG_sim8/SM_Grid_Simulation/Boost -buck Bi-directional converter 1 ==
  note: previous: OP signal
  note: DC Bus
  note: DC Bus Battery
  note: PI Controller and logic for
      | the DC/DC converter
  note: DC/DC bidirectional converter (Detailed Model)
      | Voltage Control DC/DC Bidirectional Converter for Max Demand
  note: 300V
      | Boost - Buck Converter
  1200 uF : spsSeriesRLCBranchLib/Series RLC Branch  LConnTagsString=__new0  RConnTagsString=__new0  BranchType=RC  Resistance=0.1  Inductance=3e-3  SetiL0=off  InitialCurrent=0  Capacitance=120e-6  Setx0=on  InitialVoltage=300  Measurements=None
  1200uF : spsSeriesRLCBranchLib/Series RLC Branch  LConnTagsString=__new0  RConnTagsString=__new0  BranchType=C  Resistance=1  Inductance=3e-3  SetiL0=off  InitialCurrent=0  Capacitance=1200e-6  Setx0=on  InitialVoltage=120  Measurements=None
  9mH : spsSeriesRLCBranchLib/Series RLC Branch  LConnTagsString=__new0  RConnTagsString=__new0  BranchType=L  Resistance=1  Inductance=9e-3  SetiL0=off  InitialCurrent=0  Capacitance=1e-6  Setx0=off  InitialVoltage=0  Measurements=None
  Breaker1 : spsBreakerLib/Breaker  InitialState=0  SwitchingTimes="[1/60  5/60]"  External=on  BreakerResistance=0.0001  SnubberResistance=1e6  SnubberCapacitance=inf  Measurements=None  MoreParameters=on  NoBreakLoop=off
      settings: SourceProductBaseCode=PS
  Breaker4 : spsBreakerLib/Breaker  InitialState=0  SwitchingTimes="[1/60  5/60]"  External=on  BreakerResistance=0.0001  SnubberResistance=1e6  SnubberCapacitance=inf  Measurements=None  MoreParameters=on  NoBreakLoop=off
      settings: SourceProductBaseCode=PS
  Constant : Constant
  Constant1 : Constant
  Constant2 : Constant
  Controlled Current Source : spsControlledCurrentSourceLib/Controlled Current Source  Initialize=on  Source_Type=AC  Amplitude=0  Phase=0  Frequency=0  Measurements=None
  Controlled Voltage Source : spsControlledVoltageSourceLib/Controlled Voltage Source  Initialize=on  Source_Type=DC  Amplitude=0  Phase=0  Frequency=0  Measurements=None
  Current Measurement{,2..4} (4 alike) : spsCurrentMeasurementLib/Current Measurement  PhasorSimulation=off  OutputType=Complex  PSBequivalent=0
  Display{1..3,6} (4 alike) : Display
  Divide : Product  Inputs=**/
  Divide1 : Product  Inputs=**/
  Mean : spsMeanLib/Mean  Freq=10  Vinit=0  Ts=0
  Mean1 : spsMeanLib/Mean  Freq=10  Vinit=0  Ts=0
  NOT : Logic  Operator=NOT  IconShape=distinctive  AllPortsSameDT=off  OutDataTypeStr=boolean
  Primary Control : Subsystem
      mask Display: image('Icons\FPGA.png');
  Scope : Scope
  "Two inductor inparallel 4.5 mH, 0.3 ohms" : spsSeriesRLCBranchLib/Series RLC Branch  LConnTagsString=__new0  RConnTagsString=__new0  BranchType=RL  Resistance=0.3  Inductance=4.5e-5  SetiL0=off  InitialCurrent=0  Capacitance=1e-6  Setx0=off  InitialVoltage=0  Measurements=None
  V_ref : Constant  Value=300
  "Vdc " : spsVoltageMeasurementLib/Voltage Measurement  Tag=PoWeRsYsTeMmEaSuReMeNt  PhasorSimulation=off  OutputType=Magnitude  PSBequivalent=0
  Vdc 1 : spsVoltageMeasurementLib/Voltage Measurement  Tag=PoWeRsYsTeMmEaSuReMeNt  PhasorSimulation=off  OutputType=Magnitude  PSBequivalent=0
  Voltage Measurement : spsVoltageMeasurementLib/Voltage Measurement  PhasorSimulation=off  OutputType=Complex  PSBequivalent=0
  B + : PMIOPort  Side=Right
  + : PMIOPort  Port=2  Side=Left
  - : PMIOPort  Port=3  Side=Left
  B - : PMIOPort  Port=4  Side=Right
  tag scope: I_DC_bus_BESS=global, Idc_battery=global, V_DC_bus_BESS=global, Vdc_battery=global
  wires:
  "Vdc "/1 -> Display2/1, [V_DC_bus_BESS]
  Vdc 1/1 -> Display3/1, [Vdc_battery]
  Mean/1 -> Display6/1
  Mean1/1 -> Display1/1
  V_ref/1 -> Primary Control/1(V_ref)
  Constant/1 -> NOT/1, Breaker1/1
  NOT/1 -> Breaker4/1
  Current Measurement3/1 -> Scope/1
  Voltage Measurement/1 -> [Vsec_BESS]
  Current Measurement/1 -> [Iprim_BESS]
  Primary Control/1(Duty_Ctrl) -> [Duty_Ctrl]
  Primary Control/2(Comp_Duty_Ctrl) -> [Comp_Duty_Ctrl]
  [Vsec_BESS] -> Divide/2
  Divide/1 -> Controlled Voltage Source/1
  [Comp_Duty_Ctrl] -> Divide1/1
  [Iprim_BESS] -> Divide1/2
  Divide1/1 -> Controlled Current Source/1
  [Comp_Duty_Ctrl] -> Divide/1
  Constant2/1 -> Divide/3
  Constant1/1 -> Divide1/3
  Current Measurement4/1 -> [Idc_battery], Mean1/1
  Current Measurement2/1 -> Mean/1, [I_DC_bus_BESS]
  connections:
  +/RConn1 -- Current Measurement4/LConn1 -- Vdc 1/LConn1
  Current Measurement/LConn1 -- Breaker4/LConn1 -- Breaker1/LConn1
  "Vdc "/LConn1 -- Current Measurement2/LConn1 -- 1200 uF/LConn1 -- Controlled Current Source/RConn1 -- Voltage Measurement/LConn1
  Voltage Measurement/LConn2 -- "Vdc "/LConn2 -- B -/RConn1 -- 1200 uF/RConn1 -- Controlled Voltage Source/LConn1 -- Vdc 1/LConn2 -- -/RConn1 -- 1200uF/RConn1 -- Controlled Current Source/LConn1
  "Two inductor inparallel 4.5 mH, 0.3 ohms"/LConn1 -- Breaker1/RConn1
  Current Measurement3/RConn1 -- Current Measurement4/RConn1 -- 1200uF/LConn1 -- 9mH/RConn1
  9mH/LConn1 -- Breaker4/RConn1
  "Two inductor inparallel 4.5 mH, 0.3 ohms"/RConn1 -- Current Measurement3/LConn1
  Current Measurement/RConn1 -- Controlled Voltage Source/RConn1
  Current Measurement2/RConn1 -- B +/RConn1

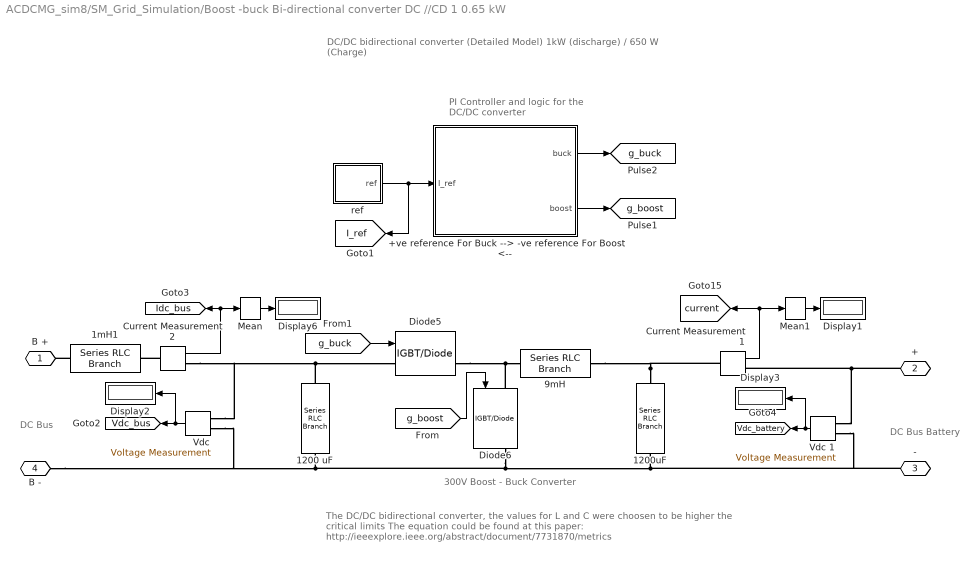
== system ACDCMG_sim8/SM_Grid_Simulation/Boost -buck Bi-directional converter DC //CD 1 0.65 kW ==
  note: DC Bus
  note: DC Bus Battery
  note: PI Controller and logic for
      | the DC/DC converter
  note: DC/DC bidirectional converter (Detailed Model)
      | 1kW (discharge) / 650 W (Charge)
  note: 300V
      | Boost - Buck Converter
  note: The DC/DC bidirectional converter, the values for L and C were choosen to be higher the critical limits The equation could be found at this paper:
      | http://ieeexplore.ieee.org/abstract/document/7731870/metrics
  +ve reference For Buck --> -ve reference For Boost <-- : Subsystem
      mask Display: image('Icons\FPGA.png');
  1200 uF : spsSeriesRLCBranchLib/Series RLC Branch  LConnTagsString=__new0  RConnTagsString=__new0  BranchType=RC  Resistance=0.1  Inductance=3e-3  SetiL0=off  InitialCurrent=0  Capacitance=1200e-6  Setx0=off  InitialVoltage=150  Measurements=None
  1200uF : spsSeriesRLCBranchLib/Series RLC Branch  LConnTagsString=__new0  RConnTagsString=__new0  BranchType=C  Resistance=1  Inductance=3e-3  SetiL0=off  InitialCurrent=0  Capacitance=1200e-6  Setx0=off  InitialVoltage=130  Measurements=None
  1mH1 : spsSeriesRLCBranchLib/Series RLC Branch  LConnTagsString=__new0  RConnTagsString=__new0  BranchType=L  Resistance=1  Inductance=1e-4  SetiL0=off  InitialCurrent=0  Capacitance=1e-6  Setx0=off  InitialVoltage=0  Measurements=None
  9mH : spsSeriesRLCBranchLib/Series RLC Branch  LConnTagsString=__new0  RConnTagsString=__new0  BranchType=L  Resistance=1  Inductance=9e-3  SetiL0=off  InitialCurrent=0  Capacitance=1e-6  Setx0=off  InitialVoltage=0  Measurements=None
  Current Measurement1 : spsCurrentMeasurementLib/Current Measurement  PhasorSimulation=off  OutputType=Complex  PSBequivalent=0
  Current Measurement2 : spsCurrentMeasurementLib/Current Measurement  PhasorSimulation=off  OutputType=Complex  PSBequivalent=0
  Diode5 : spsIGBTDiodeLib/IGBT//Diode  Ron=1e-3  Rs=1e5  Cs=inf  Measurements=on
  Diode6 : spsIGBTDiodeLib/IGBT//Diode  Ron=1e-3  Rs=1e5  Cs=inf  Measurements=on
  Display{1..3,6} (4 alike) : Display
  Mean : spsMeanLib/Mean  Freq=100  Vinit=0  Ts=0
  Mean1 : spsMeanLib/Mean  Freq=10  Vinit=0  Ts=0
  "Vdc " : spsVoltageMeasurementLib/Voltage Measurement  Tag=PoWeRsYsTeMmEaSuReMeNt  PhasorSimulation=off  OutputType=Magnitude  PSBequivalent=0
  Vdc 1 : spsVoltageMeasurementLib/Voltage Measurement  Tag=PoWeRsYsTeMmEaSuReMeNt  PhasorSimulation=off  OutputType=Magnitude  PSBequivalent=0
  ref : Subsystem
  B + : PMIOPort  Side=Right
  + : PMIOPort  Port=2  Side=Left
  - : PMIOPort  Port=3  Side=Left
  B - : PMIOPort  Port=4  Side=Right
  tag scope: I_ref=global, Idc_bus=global, Vdc_battery=global, Vdc_bus=global, current=global, g_boost=global, g_buck=global
  wires:
  "Vdc "/1 -> Display2/1, [Vdc_bus]
  Vdc 1/1 -> Display3/1, [Vdc_battery]
  Current Measurement2/1 -> Mean/1, [Idc_bus]
  [g_boost] -> Diode6/1
  +ve reference For Buck --> -ve reference For Boost <--/1(buck) -> [g_buck]
  [g_buck] -> Diode5/1
  +ve reference For Buck --> -ve reference For Boost <--/2(boost) -> [g_boost]
  Mean/1 -> Display6/1
  Current Measurement1/1 -> [current], Mean1/1
  Mean1/1 -> Display1/1
  ref/1(ref) -> [I_ref], +ve reference For Buck --> -ve reference For Boost <--/1(I_ref)
  connections:
  +/RConn1 -- Vdc 1/LConn1 -- Current Measurement1/RConn1
  9mH/LConn1 -- Diode5/RConn1 -- Diode6/LConn1
  1200 uF/LConn1 -- "Vdc "/LConn1 -- Current Measurement2/RConn1 -- Diode5/LConn1
  1200uF/LConn1 -- Current Measurement1/LConn1 -- 9mH/RConn1
  Diode6/RConn1 -- "Vdc "/LConn2 -- B -/RConn1 -- 1200 uF/RConn1 -- Vdc 1/LConn2 -- -/RConn1 -- 1200uF/RConn1
  Current Measurement2/LConn1 -- 1mH1/RConn1
  1mH1/LConn1 -- B +/RConn1

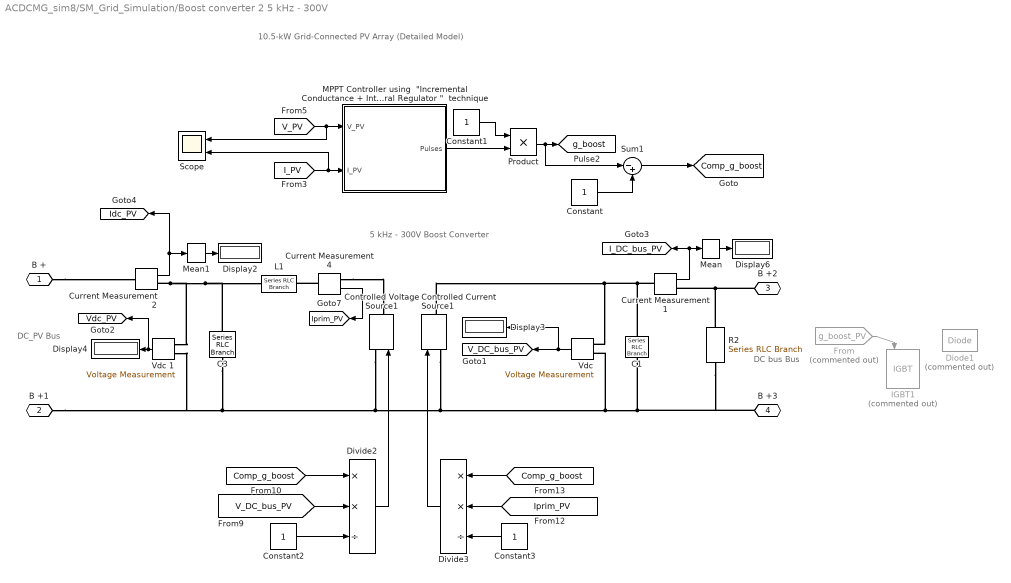
== system ACDCMG_sim8/SM_Grid_Simulation/Boost converter 2 5 kHz - 300V  ==
  note: DC_PV Bus
  note: DC bus Bus
  note: 5 kHz - 300V
      | Boost Converter
  note: 10.5-kW Grid-Connected PV Array (Detailed Model)
  C1 : spsSeriesRLCBranchLib/Series RLC Branch  LConnTagsString=__new0  RConnTagsString=__new0  BranchType=C  Resistance=1.0  Inductance=1.0  SetiL0=off  InitialCurrent=0  Capacitance=6000e-06  Setx0=off  InitialVoltage=0  Measurements=None
  C3 : spsSeriesRLCBranchLib/Series RLC Branch  LConnTagsString=__new0  RConnTagsString=__new0  BranchType=C  Resistance=1.0  Inductance=1.0  SetiL0=off  InitialCurrent=0  Capacitance=100e-6  Setx0=off  InitialVoltage=0  Measurements=Branch voltage
  Constant{,1..3} (4 alike) : Constant
  Controlled Current Source1 : spsControlledCurrentSourceLib/Controlled Current Source  Initialize=on  Source_Type=AC  Amplitude=0  Phase=0  Frequency=0  Measurements=None
  Controlled Voltage Source1 : spsControlledVoltageSourceLib/Controlled Voltage Source  Initialize=on  Source_Type=DC  Amplitude=0  Phase=0  Frequency=0  Measurements=None
  Current Measurement1 : spsCurrentMeasurementLib/Current Measurement  PhasorSimulation=off  OutputType=Complex  PSBequivalent=0
  Current Measurement2 : spsCurrentMeasurementLib/Current Measurement  PhasorSimulation=off  OutputType=Complex  PSBequivalent=0
  Current Measurement4 : spsCurrentMeasurementLib/Current Measurement  PhasorSimulation=off  OutputType=Complex  PSBequivalent=0
  Diode1 : spsDiodeLib/Diode  Commented=on  Ron=1e-4  Lon=0  Vf=0  IC=0  UseSnubber=off  Rs=inf  Cs=inf  Measurements=off
  Display{2..4,6} (4 alike) : Display
  Divide2 : Product  Inputs=**/
  Divide3 : Product  Inputs=**/
  From : From  Commented=on  GotoTag=g_boost_PV  TagVisibility=global
  IGBT1 : spsIGBTLib/IGBT  Commented=on  Ron=0.001  Lon=0  Vf=0  Tf=0  Tt=0  IC=0  Rs=1e5  Cs=inf  Measurements=off
  L1 : spsSeriesRLCBranchLib/Series RLC Branch  LConnTagsString=__new0  RConnTagsString=__new0  BranchType=RL  Resistance=0.005  Inductance=5e-3  SetiL0=off  InitialCurrent=0  Capacitance=1e-6  Setx0=off  InitialVoltage=0  Measurements=None
  "MPPT Controller using  \"Incremental Conductance + Integral Regulator \"  technique " : Subsystem  mask(Boost Control - MPPT){fc=5000, T_MPPT=200e-6, Dinit=0.3}
      mask prompts: fc "PWM switching frequency (Hz)"; T_MPPT "Time window used by MPPT control (s)"; Dinit "Initial value of duty cycle"
      mask Display: image('Icons\FPGA.png');
  Mean : spsMeanLib/Mean  Freq=1000  Vinit=0  Ts=0
  Mean1 : spsMeanLib/Mean  Freq=5000  Vinit=0  Ts=Ts_Power
  Product : Product
  R2 : spsSeriesRLCBranchLib/Series RLC Branch  LConnTagsString=__new0  RConnTagsString=__new0  BranchType=R  Resistance=1000  Inductance=5e-3  SetiL0=off  InitialCurrent=0  Capacitance=1e-6  Setx0=off  InitialVoltage=0  Measurements=None
  Scope : Scope  NumInputPorts=2
  Sum1 : Sum  Inputs=|-+
  "Vdc " : spsVoltageMeasurementLib/Voltage Measurement  Tag=PoWeRsYsTeMmEaSuReMeNt  PhasorSimulation=off  OutputType=Magnitude  PSBequivalent=0
  Vdc 1 : spsVoltageMeasurementLib/Voltage Measurement  Tag=PoWeRsYsTeMmEaSuReMeNt  PhasorSimulation=off  OutputType=Magnitude  PSBequivalent=0
  B + : PMIOPort  Side=Right
  B +1 : PMIOPort  Port=2  Side=Right
  B +2 : PMIOPort  Port=3  Side=Right
  B +3 : PMIOPort  Port=4  Side=Right
  tag scope: Comp_g_boost=global, I_DC_bus_PV=global, Idc_PV=global, Iprim_PV=global, V_DC_bus_PV=global, Vdc_PV=global, g_boost=global
  wires:
  [I_PV] -> Scope/2, "MPPT Controller using  \"Incremental Conductance + Integral Regulator \"  technique "/2(I_PV)
  "MPPT Controller using  \"Incremental Conductance + Integral Regulator \"  technique "/1(Pulses) -> Product/2
  [V_PV] -> Scope/1, "MPPT Controller using  \"Incremental Conductance + Integral Regulator \"  technique "/1(V_PV)
  Constant1/1 -> Product/1
  Current Measurement2/1 -> [Idc_PV], Mean1/1
  Mean/1 -> Display6/1
  Current Measurement1/1 -> [I_DC_bus_PV], Mean/1
  "Vdc "/1 -> Display3/1, [V_DC_bus_PV]
  Vdc 1/1 -> [Vdc_PV], Display4/1
  Mean1/1 -> Display2/1
  From/1 -> IGBT1/1
  Current Measurement4/1 -> [Iprim_PV]
  [V_DC_bus_PV] -> Divide2/2
  Divide2/1 -> Controlled Voltage Source1/1
  Constant2/1 -> Divide2/3
  [Comp_g_boost] -> Divide2/1
  [Comp_g_boost] -> Divide3/1
  Constant3/1 -> Divide3/3
  [Iprim_PV] -> Divide3/2
  Divide3/1 -> Controlled Current Source1/1
  Product/1 -> Sum1/1, [g_boost]
  Sum1/1 -> [Comp_g_boost]
  Constant/1 -> Sum1/2
  connections:
  Current Measurement2/RConn1 -- Vdc 1/LConn1 -- L1/LConn1 -- C3/LConn1
  C3/RConn1 -- Controlled Voltage Source1/LConn1 -- Controlled Current Source1/LConn1 -- R2/LConn1 -- B +3/RConn1 -- C1/RConn1 -- "Vdc "/LConn2 -- B +1/RConn1 -- Vdc 1/LConn2
  Current Measurement4/LConn1 -- L1/RConn1
  B +/RConn1 -- Current Measurement2/LConn1
  B +2/RConn1 -- R2/RConn1 -- Current Measurement1/RConn1
  C1/LConn1 -- Current Measurement1/LConn1 -- Controlled Current Source1/RConn1 -- "Vdc "/LConn1
  Current Measurement4/RConn1 -- Controlled Voltage Source1/RConn1
